simulink model "Q3_Mean_Std"  (R2024b)
settings: Solver=VariableStepAuto  StartTime=0.0  StopTime=10.0  RelTol=1e-3
model workspace (MAT data in the model file):
  input_array = [0; 1.2; 2.4; 3.6; 4.8; 6; 7.2; 8.4; 9.6; 10.8; 12; 13.2; 14.4; 15.6; 16.8; 18; 19.2; 20.4; 21.6; 22.8; 24; 25.2; 26.4; 27.6; 28.8; 30]
settings Model: Creator=chall  LastModifiedBy=chall
settings RTWCC: GPUComputeCapability=3.5

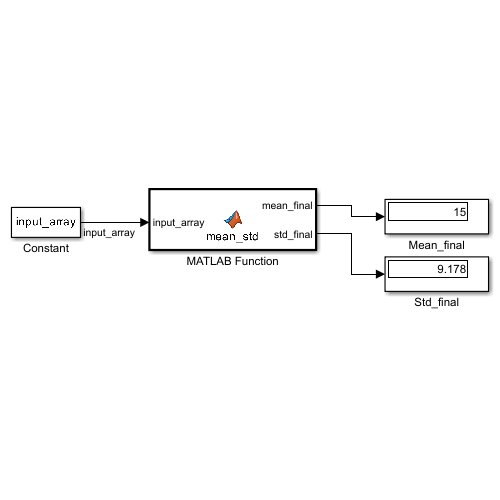
[thumbnail: Simulink's stored preview of the top-level diagram]
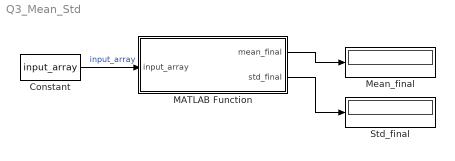
== system Q3_Mean_Std ==
  Constant : Constant  Value=input_array
  MATLAB Function : MATLAB Function  TreatAsAtomicUnit=on
  Mean_final : Display
  Std_final : Display
  wires:
  Constant/1 -> MATLAB Function/1(input_array)  "input_array"
  MATLAB Function/1(mean_final) -> Mean_final/1
  MATLAB Function/2(std_final) -> Std_final/1

== matlab function Q3_Mean_Std/MATLAB Function ==
  data: input_array input; mean_final output; std_final output
function [mean_final,std_final] = mean_std(input_array)

mean_final = mean(input_array);
std_final = std(input_array);
end
